simulink model "etc5d"  (Simulink 5.0)
settings: Solver=ode15s  StartTime=0.0  StopTime=0.5  FixedStep=1e-3  RelTol=1e-5  AbsTol=1e-8
PreLoadFcn:
  | setup5d,etc_def
values from neighbouring files (symbols this model uses):
  alpha_des = (pi/2)*(89.8/90)    (= 1.56730566829)    [etc_def.m]
  surfA = lambda*(alpha-ufA)+(omega-ufdotA)    [etc_def.m]
  surfB = -lambda*ufB-ufdotB    [etc_def.m]
undefined symbols (not defined in the file or in its folder): red_fil
libraries: cmlib x10
settings Model: LastModifiedBy=ansgar  ExtModeTrigMode=oneshot  ExtModeArmWhenConnect=off  LimitDataPoints=off  BlockReductionOpt=off

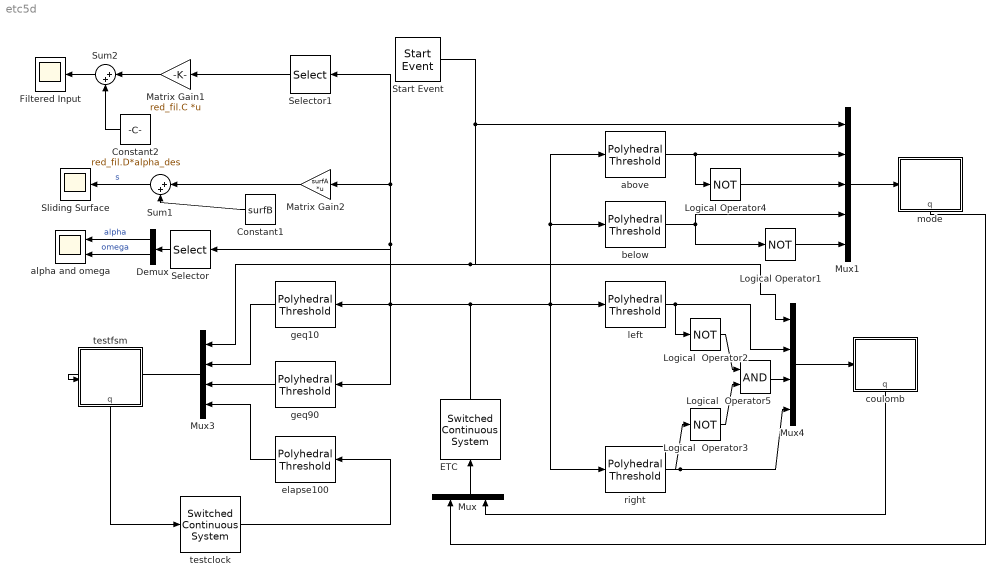
== system etc5d ==
  Constant1 : Constant  Orientation=left  Value=surfB
  Constant2 : Constant  Orientation=left  Value=red_fil.D*alpha_des
  Demux : Demux  Orientation=left  Outputs=2
  ETC : cmlib/Switched Continuous System  Orientation=up  AncestorBlock=cmlib/Switched Continuous System  nx=4  use_sd=off  nup=[]  nz=[]  use_reset=off  nu=2  x0=[0;0;0;0]  swfunc=slidingmode  ICS=etc_ICS  AR=etc_AR  use_param=on  p0=[1.2;1.2]  PaCs=etc_PaCs
  Filtered Input : Scope
      settings: TimeRange=0.5  YMin=-0.5  YMax=2
  Logical  Operator2 : Logic  Operator=NOT
  Logical  Operator3 : Logic  Operator=NOT
  Logical  Operator5 : Logic
  Logical Operator1 : Logic  Operator=NOT
  Logical Operator4 : Logic  Operator=NOT
  Matrix Gain1 : Gain  Orientation=left  Gain=red_fil.C  Multiplication=Matrix(K*u)  SaturateOnIntegerOverflow=on
  Matrix Gain2 : Gain  Orientation=left  Gain=surfA  Multiplication=Matrix(K*u)  SaturateOnIntegerOverflow=on
  Mux : Mux  Orientation=up  Inputs=2
  Mux1 : Mux  Inputs=5
  Mux3 : Mux  Orientation=left
  Mux4 : Mux
  Selector : Selector  Orientation=left  Elements=[3 4]  InputPortWidth=4
  Selector1 : Selector  Orientation=left  Elements=[1 2]  InputPortWidth=4
  Sliding Surface : Scope
      settings: TimeRange=0.5  YMax=35  SaveName=ScopeData4
  Start Event : cmlib/Start Event  steptime=0.01  initval=0  finival=1  sampletime=0  interpret=on  enable=on
  Sum1 : Sum  Orientation=left  Inputs=|++  SaturateOnIntegerOverflow=on  InputSameDT=on
  Sum2 : Sum  Orientation=left  Inputs=|++  SaturateOnIntegerOverflow=on  InputSameDT=on
  above : cmlib/Polyhedral Threshold  polyhedron=above_surf
  alpha and omega : Scope  NumInputPorts=2
      settings: TimeRange=0.5  YMin=0~-10  YMax=2~30  SaveName=AandO  DataFormat=Structure
  below : cmlib/Polyhedral Threshold  polyhedron=below_surf
  coulomb : Stateflow chart  Orientation=down  TreatAsAtomicUnit=on
  elapse100 : cmlib/Polyhedral Threshold  Orientation=left  polyhedron=clock_geq100
  geq10 : cmlib/Polyhedral Threshold  Orientation=left  polyhedron=alpha_geq10
  geq90 : cmlib/Polyhedral Threshold  Orientation=left  polyhedron=alpha_geq90
  left : cmlib/Polyhedral Threshold  polyhedron=turn_left
  mode : Stateflow chart  Orientation=down  TreatAsAtomicUnit=on
  right : cmlib/Polyhedral Threshold  polyhedron=turn_right
  testclock : cmlib/Switched Continuous System  AncestorBlock=cmlib/Switched Continuous System  nx=1  use_sd=off  nup=[]  nz=[]  use_reset=off  nu=1  x0=0  swfunc=testclock  ICS=clock_ICS  AR=clock_AR  use_param=off  p0=[]  PaCs=[]
  testfsm : Stateflow chart  Orientation=down  TreatAsAtomicUnit=on
  wires:
  ETC/1 -> left/1, below/1, above/1, right/1, geq90/1, Matrix Gain2/1, Selector1/1, Selector/1, geq10/1
  Mux/1 -> ETC/1
  mode/1(q) -> Mux/1
  Matrix Gain2/1 -> Sum1/1
  Constant1/1 -> Sum1/2
  Sum1/1 -> Sliding Surface/1  "s"
  Mux4/1 -> coulomb/Trigger
  left/1 -> Mux4/2, Logical  Operator2/1
  right/1 -> Mux4/4, Logical  Operator3/1
  Mux1/1 -> mode/Trigger
  Logical Operator1/1 -> Mux1/5
  Logical Operator4/1 -> Mux1/3
  below/1 -> Logical Operator1/1, Mux1/4
  above/1 -> Logical Operator4/1, Mux1/2
  coulomb/1(q) -> Mux/2
  Start Event/1 -> Mux1/1, Mux4/1, Mux3/1
  Selector/1 -> Demux/1
  Demux/1 -> alpha and omega/1  "alpha"
  Demux/2 -> alpha and omega/2  "omega"
  Selector1/1 -> Matrix Gain1/1
  Sum2/1 -> Filtered Input/1
  Matrix Gain1/1 -> Sum2/1
  Constant2/1 -> Sum2/2
  testclock/1 -> elapse100/1
  Mux3/1 -> testfsm/Trigger
  testfsm/1(q) -> testclock/1
  geq10/1 -> Mux3/2
  geq90/1 -> Mux3/3
  elapse100/1 -> Mux3/4
  Logical  Operator5/1 -> Mux4/3
  Logical  Operator2/1 -> Logical  Operator5/1
  Logical  Operator3/1 -> Logical  Operator5/2

== stateflow chart mode ==
  state on
    entry: q=1;
  state under
    entry: q=2;
  state beyond
    entry: q=3;
  on -> under : below
  on -> beyond : above
  under -> on : negbelow
  (default) -> beyond : start
  beyond -> on : negabove
  data: q output int16
  events: start input RISING_EDGE_EVENT; above input RISING_EDGE_EVENT; negabove input RISING_EDGE_EVENT; below input RISING_EDGE_EVENT; negbelow input RISING_EDGE_EVENT

== stateflow chart testfsm ==
  state above0
    entry: q=1;
  state above10
    entry:q=2;
  state reach
    entry: q=4;
  state avoid
    entry: q=3;
  (default) -> above0 : start
  above0 -> above10 : geq10
  above10 -> reach : geq90
  above10 -> avoid : elapse100
  data: q output int16
  events: start input RISING_EDGE_EVENT; geq10 input RISING_EDGE_EVENT; geq90 input RISING_EDGE_EVENT; elapse100 input RISING_EDGE_EVENT

== stateflow chart coulomb ==
  state left
    entry: q=2;
  state right
    entry: q=3;
  state neither
    entry: q=1;
  left -> neither : negturn
  (default) -> neither : start
  right -> neither : negturn
  neither -> right : turnright
  neither -> left : turnleft
  data: q output int16
  events: start input RISING_EDGE_EVENT; turnleft input RISING_EDGE_EVENT; negturn input RISING_EDGE_EVENT; turnright input RISING_EDGE_EVENT
